simulink model "PendCart"  (R2024b)
settings: Solver=ode45  StartTime=0.0  StopTime=4  FixedStep=0.001  MaxStep=0.005  RelTol=1e-3
libraries: simulink x2
settings Model: Creator=mattf  LastModifiedBy=benva
settings DataIOCC: SaveFinalState=on  SaveOperatingPoint=on

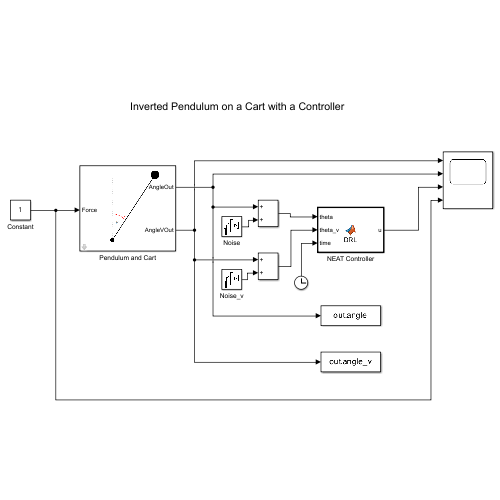
[thumbnail: Simulink's stored preview of the top-level diagram]
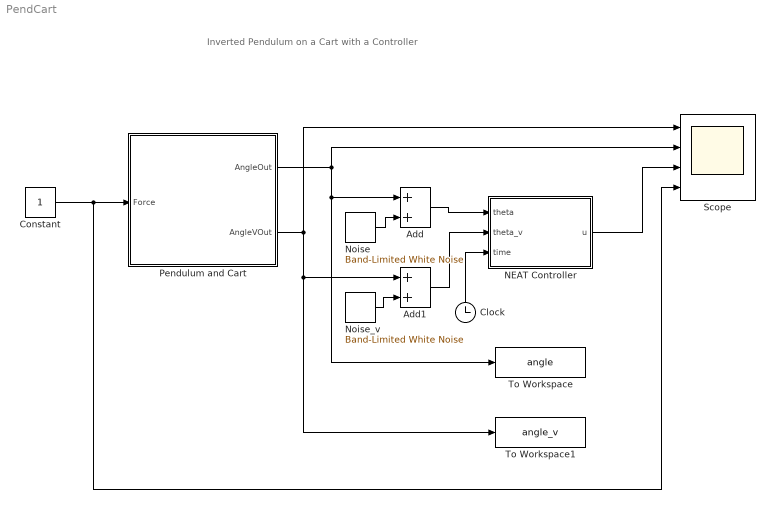
== system PendCart ==
  note: Inverted Pendulum on a Cart with a Controller
  Add : Sum
  Add1 : Sum
  Clock : Clock
  Constant : Constant
  NEAT Controller : MATLAB Function  TreatAsAtomicUnit=on
  Noise : simulink/Sources/Band-Limited White Noise  Cov=[0]  Ts=0.001  seed=[7555]
  Noise_v : simulink/Sources/Band-Limited White Noise  Cov=[0]  Ts=0.001  seed=[35347]
  Pendulum and Cart : Subsystem  mask{Mcart=0.5, m=0.2, l=0.3/2, g=9.8, init=0.889113259339537}
      mask prompts: Mcart "Cart Mass (kg):"; m "Pend Mass (kg):"; l "COM Distance (m):"; g "Acc due to Gravity (g):"; init "Initial Angle (rad):"
      mask Display: image('pen img.png');
  Scope : Scope  NumInputPorts=4
  To Workspace : ToWorkspace  VariableName=angle  SampleTime=-1
  To Workspace1 : ToWorkspace  VariableName=angle_v  SampleTime=-1
  wires:
  Pendulum and Cart/2(AngleVOut) -> Add1/1, To Workspace1/1, Scope/1
  Clock/1 -> NEAT Controller/3(time)
  Pendulum and Cart/1(AngleOut) -> Add/1, To Workspace/1, Scope/2
  Add/1 -> NEAT Controller/1(theta)
  Noise/1 -> Add/2
  Noise_v/1 -> Add1/2
  Add1/1 -> NEAT Controller/2(theta_v)
  Constant/1 -> Pendulum and Cart/1(Force), Scope/4
  NEAT Controller/1(u) -> Scope/3

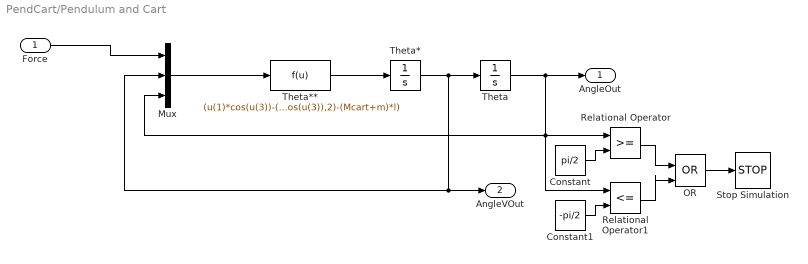
== system PendCart/Pendulum and Cart ==
  Force : Inport
  Constant : Constant  Value=pi/2
  Constant1 : Constant  Value=-pi/2
  Mux : Mux  Inputs=3
  OR : Logic  Operator=OR  IconShape=distinctive  AllPortsSameDT=off  OutDataTypeStr=boolean
  Relational Operator : RelationalOperator  OutDataTypeStr=boolean  RndMeth=Simplest  InputSameDT=off
  Relational Operator1 : RelationalOperator  Operator=<=  OutDataTypeStr=boolean  RndMeth=Simplest  InputSameDT=off
  Stop Simulation : Stop
  Theta : Integrator  InitialCondition=init
  Theta* : Integrator
  Theta** : Fcn  Expr=(u(1)*cos(u(3))-(Mcart+m)*g*sin(u(3))+m*l*cos(u(3))*sin(u(3))*power(u(2),2))/(m*l*power(cos(u(3)),2)-(Mcart+m)*l)
  AngleOut : Outport
  AngleVOut : Outport  Port=2
  wires:
  Mux/1 -> Theta**/1
  Theta**/1 -> Theta*/1
  Theta*/1 -> Mux/2, AngleVOut/1, Theta/1
  Theta/1 -> AngleOut/1, Relational Operator1/1, Relational Operator/1, Mux/3
  Constant/1 -> Relational Operator/2
  Constant1/1 -> Relational Operator1/2
  OR/1 -> Stop Simulation/1
  Relational Operator1/1 -> OR/2
  Relational Operator/1 -> OR/1
  Force/1 -> Mux/1

== matlab function PendCart/NEAT Controller ==
  settings: updateMethod=CONTINUOUS
  data: u output; theta input; theta_v input; time input
function u = DRL(theta, theta_v, time)
%#codegen
    %--- declare extrinsic calls ---
    coder.extrinsic('py.drl_controller.controller_call');
    %coder.extrinsic('disp','num2str');
    
    %--- get your u from Python as before ---
    u = coder.nullcopy(zeros(1,1));
    u = double(py.drl_controller.controller_call(theta, theta_v, time));

    %--- print it ---
    %disp([ 'DRL:: u = ' num2str(u) ]);
end
